simulink model "untitled"  (R2018b)
settings: Solver=VariableStepAuto  StartTime=0.0  StopTime=5  RelTol=1e-3
libraries: dsparch4 x1, dspsigops x1
settings Model: Creator=nhat  LastModifiedBy=nhat

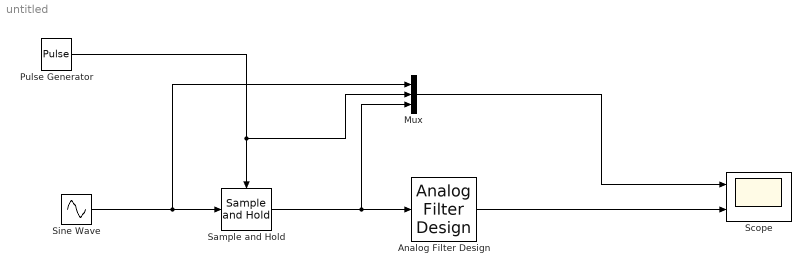
== system untitled ==
  Analog Filter Design : dsparch4/Analog Filter Design  method=Butterworth  filttype=Lowpass  N=8  Wlo=3100*pi*2  Whi=80  Rp=2  Rs=40
  Mux : Mux  Inputs=3
  Pulse Generator : DiscretePulseGenerator  PulseType=Time based  Period=1/8000  PulseWidth=50
  Sample and Hold : dspsigops/Sample and Hold  trig=Rising edge  initCond=0  latchinput=off
  Scope : Scope  NumInputPorts=2
  Sine Wave : Sin  Frequency=3000*2*pi  SampleTime=1/64000
  wires:
  Sine Wave/1 -> Mux/1, Sample and Hold/1
  Pulse Generator/1 -> Mux/2, Sample and Hold/Trigger
  Sample and Hold/1 -> Mux/3, Analog Filter Design/1
  Analog Filter Design/1 -> Scope/2
  Mux/1 -> Scope/1
